simulink model "coagul_m"  (Simulink 8.5)
settings: Solver=ode45  SolverMode=SingleTasking  StartTime=0.0  StopTime=999999  MaxStep=10  RelTol=1e-3  AbsTol=1e-3
values from neighbouring files (symbols this model uses):
  U = st_Varia('LongNames')    [coagul_i.m]
  x0 = []    [coagul_i.m]    (also in coagul_s.m = x0)
undefined symbols (not defined in the file or in its folder): B
settings Model: Creator=psross  LastModifiedBy=Martijn
settings DataIOCC: LimitDataPoints=off  SaveOutput=off  SaveTime=off  SignalLoggingName=sigsOut
settings OptimizationCC: BooleanDataType=off
settings DebuggingCC: SaveWithParameterizedLinksMsg=none  SignalResolutionControl=TryResolveAllWithWarning  MultiTaskDSMMsg=warning  MultiTaskCondExecSysMsg=none  FcnCallInpInsideContextMsg=UseLocalSettings  StrictBusMsg=None
settings HardwareCC: TargetUnknown=on

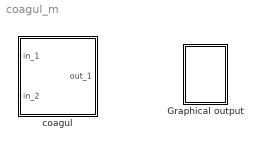
== system coagul_m ==
  Graphical output : Subsystem
      settings: OpenFcn=coagul_g
      mask Display:
      | plot(0,0,100,100,[80,20,20],[20,20,80],[80,69,60,52,45,39,33,28,24,20],[65,65,64,61,57,52,45,37,30,20])
      | disp('');
      | text(100,100,'coagul', 'horizontalAlignment', 'right', 'verticalAlignment', 'top');
  coagul : Subsystem  Description=This model calculates the removal of suspended solids with a flocculation reactor.
      mask init:
      | filenaam='.\StimelaData\Flocculation.mat';
      | 
      | [Pn,Fn,Fext]=Fileprop(filenaam);
      | 
      | errstr = st_UniqName(filenaam,'filenaam=''','SubSystem','OpenFcn');
      | if errstr, error([errstr 'The filename "' filenaam '" is already in use. Choose a different filename.']), end
      | 
      | P = coagul_p(filenaam);
      | [B,x0,U]=coagul_i(filenaam);
      | V = st_Varia;
      settings: OpenFcn=|
      | filenaam='.\StimelaData\Flocculation.mat';
      | st_ParameterInput('init',gcb,filenaam,'coagul');
      mask Display:
      | plot(0,0,100,100,[80,80,20,20],[80,20,20,80],[80,20],[70,70],[50,50],[90,40],[50,61,65,67,69,70,70,69,67,65,61,50],[40,46,47,47,45,42,38,35,33,33,34,40],[50,39,35,33,31,30,30,31,33,35,39,50],[40,46,47,47,45,42,38,35,33,33,34,40])
      | disp('')
      | text(50,50,'coagul', 'horizontalAlignment', 'center', 'verticalAlignment', 'middle');
      | text(50,0,Fn, 'horizontalAlignment', 'center', 'verticalAlignment', 'base');

== system coagul_m/Graphical output ==
  note: plotten

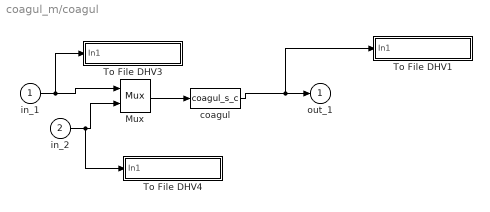
== system coagul_m/coagul ==
  in_1 : Inport
  in_2 : Inport  Port=2
  Mux : Mux  Inputs=[U.Number B.Setpoints]
  To File DHV1 : Subsystem  mask(To File DHV){naam=[filenaam(1:length(filenaam)-4) '_out.sti']}
      mask prompts: naam "Naam van bestand"
      mask init:
      | set_param([gcb '/To File'],'Filename',naam);
      mask Display: disp(naam)
  To File DHV3 : Subsystem  mask(To File DHV){naam=[filenaam(1:length(filenaam)-4) '_in.sti']}
      mask prompts: naam "Naam van bestand"
      mask init:
      | set_param([gcb '/To File'],'Filename',naam);
      mask Display: disp(naam)
  To File DHV4 : Subsystem  mask(To File DHV){naam=[filenaam(1:length(filenaam)-4) '_ES.sti']}
      mask prompts: naam "Naam van bestand"
      mask init:
      | set_param([gcb '/To File'],'Filename',naam);
      mask Display: disp(naam)
  coagul : S-Function  FunctionName=coagul_s_c  Parameters=B,x0,U,P
  out_1 : Outport  InitialOutput=0
  wires:
  in_2/1 -> To File DHV4/1(In1), Mux/2
  in_1/1 -> To File DHV3/1(In1), Mux/1
  Mux/1 -> coagul/1
  coagul/1 -> To File DHV1/1(In1), out_1/1

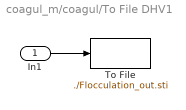
== system coagul_m/coagul/To File DHV1 ==
  In1 : Inport
  To File : ToFile  Filename=./Flocculation_out.sti  MatrixName=coagulout
  wires:
  In1/1 -> To File/1

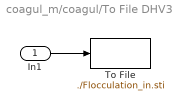
== system coagul_m/coagul/To File DHV3 ==
  In1 : Inport
  To File : ToFile  Filename=./Flocculation_in.sti  MatrixName=coagulin
  wires:
  In1/1 -> To File/1

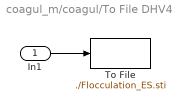
== system coagul_m/coagul/To File DHV4 ==
  In1 : Inport
  To File : ToFile  Filename=./Flocculation_ES.sti  MatrixName=coagulES
  wires:
  In1/1 -> To File/1
